simulink model "Demo_V2X_RoadWorks_cs"  (R2014b)
settings: Solver=ode5  SolverMode=SingleTasking  StartTime=0.0  StopTime=18  FixedStep=1/100  RelTol=1e-3
PreLoadFcn:
  | mbxruntime.callbacks.PreLoadFcn(bdroot);
  | check_NUTS_defined;
  | 
  | assignin('base',['model_closed_' bdroot],false);
PostLoadFcn:
  | mbxruntime.callbacks.PostLoadFcn(bdroot);
InitFcn:
  | mbxruntime.callbacks.InitFcn(bdroot);
StartFcn:
  | mbxruntime.callbacks.StartFcn(bdroot);
StopFcn:
  | mbxruntime.callbacks.StopFcn(bdroot);
model workspace: external: MAT-File .\Demo_V2X_RoadWorks_cs_hws.mat (data not in the file)
undefined symbols (not defined in the file or in its folder): InitializeBus, mbxruntime, Newton, Raphson, tabledata
undefined symbols (not defined in the file): Demo_V2X_RoadWorks_cs_002408181c311178, Demo_V2X_RoadWorks_cs_02afd40c5576fd79, Demo_V2X_RoadWorks_cs_09062d95c4976b80, Demo_V2X_RoadWorks_cs_0ad60e46608f1bfe, Demo_V2X_RoadWorks_cs_0b386a01b2cd5e8d, Demo_V2X_RoadWorks_cs_0d795afaa024d2ee, Demo_V2X_RoadWorks_cs_104085e65c337077, Demo_V2X_RoadWorks_cs_126564f7b2997a49, Demo_V2X_RoadWorks_cs_15e6e2595e8bf329, Demo_V2X_RoadWorks_cs_16adfea7655bce18, Demo_V2X_RoadWorks_cs_18ab2686f8449f50, Demo_V2X_RoadWorks_cs_1c28437def32f9f6, Demo_V2X_RoadWorks_cs_1d541c73c3d8f25b, Demo_V2X_RoadWorks_cs_1fb1f994fe012d27, Demo_V2X_RoadWorks_cs_20c117b9827230b9, Demo_V2X_RoadWorks_cs_220b1226a84e3b37, Demo_V2X_RoadWorks_cs_24814049c8ab2e18, Demo_V2X_RoadWorks_cs_24a281220a6492a7, Demo_V2X_RoadWorks_cs_279aea126b4236ad, Demo_V2X_RoadWorks_cs_28eadd0b23e572db, Demo_V2X_RoadWorks_cs_291fe7210f9ba434, Demo_V2X_RoadWorks_cs_2fd90504f8814746, Demo_V2X_RoadWorks_cs_33c1737bfc1c651f, Demo_V2X_RoadWorks_cs_388e22d5b1056b8f, Demo_V2X_RoadWorks_cs_3e3a415e868663e7, Demo_V2X_RoadWorks_cs_45759eb0c1816b1e, Demo_V2X_RoadWorks_cs_45f301cf6c396570, Demo_V2X_RoadWorks_cs_47686124f5151dea, Demo_V2X_RoadWorks_cs_487931e8a8cef1d6, Demo_V2X_RoadWorks_cs_54cb5626dca53ab7, Demo_V2X_RoadWorks_cs_56c0a253fe7e7ec0, Demo_V2X_RoadWorks_cs_5921488c0ba4168e, Demo_V2X_RoadWorks_cs_5ca0c70551eea1b3, Demo_V2X_RoadWorks_cs_5cc6ddb60eb17926, Demo_V2X_RoadWorks_cs_5dda33a127b53dd9, Demo_V2X_RoadWorks_cs_60729aca19e3b8ea, Demo_V2X_RoadWorks_cs_61616eaaf58ec115, Demo_V2X_RoadWorks_cs_63af626c9fae5224, Demo_V2X_RoadWorks_cs_649c6af7b111a61f, Demo_V2X_RoadWorks_cs_64e2df335ac415c1, Demo_V2X_RoadWorks_cs_6530f1ae727e39fe, Demo_V2X_RoadWorks_cs_6837be8d052ff1e3, Demo_V2X_RoadWorks_cs_6e8b51a123f1a201, Demo_V2X_RoadWorks_cs_6f4ec518a68cacb3, Demo_V2X_RoadWorks_cs_74dac4a6b9859226, Demo_V2X_RoadWorks_cs_75671d8cae67d5b6, Demo_V2X_RoadWorks_cs_756d40a88ae84d39, Demo_V2X_RoadWorks_cs_77c7cbc4fa1cdaa5, Demo_V2X_RoadWorks_cs_7b9fbc44403bb8f3, Demo_V2X_RoadWorks_cs_7c118b74c8d14c00, Demo_V2X_RoadWorks_cs_7c4a172761f05beb, Demo_V2X_RoadWorks_cs_80b7a78efe24d5f1, Demo_V2X_RoadWorks_cs_82d65efce1f7c4ea, Demo_V2X_RoadWorks_cs_8be5dc2565229ce9, Demo_V2X_RoadWorks_cs_8dc36f0ab6cec640, Demo_V2X_RoadWorks_cs_91305dd1362bb00d, Demo_V2X_RoadWorks_cs_929c2ffed1faf33f, Demo_V2X_RoadWorks_cs_95615bcbc0d062f1, Demo_V2X_RoadWorks_cs_99a6391a40f894df, Demo_V2X_RoadWorks_cs_9caa19175765ea5d ... (+52)
libraries: PreScanSimulinkLibrary x34, simulink_extras x15, simulink x6
(part 1 of 16)
CloseFcn:
  | mbxruntime.callbacks.CloseFcn(bdroot);
  | evalin('base',['clear model_closed_' bdroot]);
  | 
  | try
  |     close (V2x_TC_GUI)
  | end
settings Model: Creator=PRESCAN  LastModifiedBy=stq0ee
settings DataIOCC: SignalLoggingSaveFormat=ModelDataLogs
settings OptimizationCC: InlineParams=on  ExpressionDepthLimit=2147483647  InitFltsAndDblsToZero=on
settings DebuggingCC: SaveWithParameterizedLinksMsg=none  UnderspecifiedInitializationDetection=Classic  MergeDetectMultiDrivingBlocksExec=none  SignalResolutionControl=TryResolveAllWithWarning  SolverPrmCheckMsg=none  MultiTaskDSMMsg=warning  MultiTaskCondExecSysMsg=none  FcnCallInpInsideContextMsg=UseLocalSettings  StateNameClashWarn=warning
settings ModelReferenceCC: UpdateModelReferenceTargets=IfOutOfDate
settings SFSimCC: SimParseCustomCode=off
settings SFSimCC: SimCustomHeaderCode=|
  | #include "prescan.h"
  | #include "prescan_platform.h"
  | #include "prescan_v2x_data.h"
settings RTWCC: IncludeERTFirstTime=on
settings GRTTargetCC: TargetFcnLib=ansi_tfl_tmw.mat  CombineOutputUpdateFcns=off  GRTInterface=on

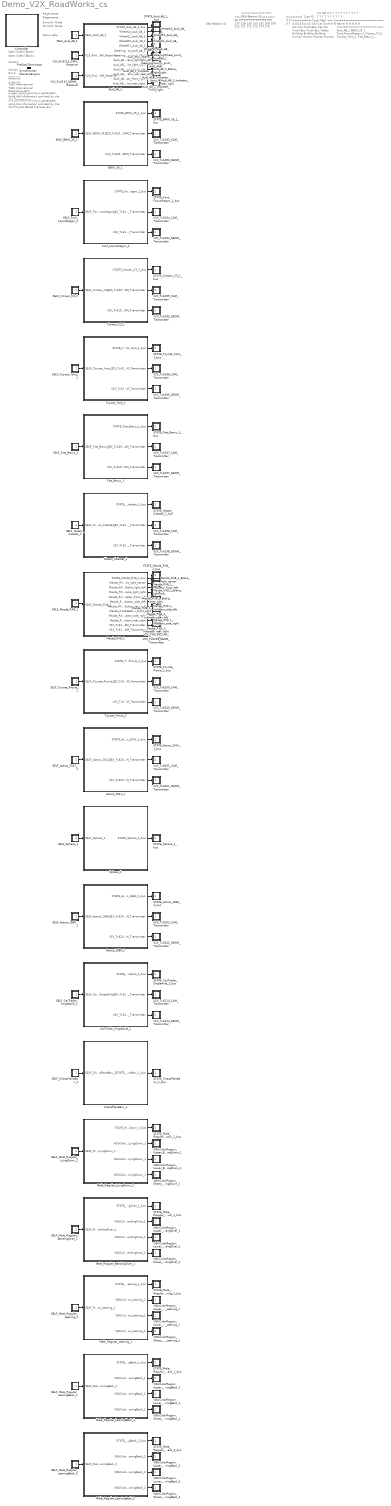
== system Demo_V2X_RoadWorks_cs ==
  note: Regenerate
  note: Simulink Mode
  note: Open Useful Blocks
  note: 2020.1.0
  note: Version:
  note: Author(s):
  note: TASS International
  note: Descriptive text:
  note: A road works warning is generated
      | using the information provided by
      | the V2X Physics Based Transceivers.
  note: OBU-Beacon ID
  note: Demo Help
  note: 8.6.0
  note: A road works warning is generated
      | using the information provided by
      | the V2X Transceivers.
  note: Descriptive text:
  note: TASS International
  note: Author(s):
  note: Version:
  note: Open Useful Blocks
  note: Simulink Mode
  note: Regenerate
  note: ======
      | Num ID
      | ======
      | 36
      | 95
      | 130
      | 131
      | 132
      | 133
      | 135
      | 137
      | 138
      | 139
      | 153
      | 152
      | 208
      | 209
      | 212
      | 171
      | 172
      | 173
      | 174
      | 175
  note: =============
      | OBU-Beacon ID
      | =============
  note: =======
      | Type ID
      | =======
      | 1
      | 1
      | 1
      | 1
      | 1
      | 1
      | 3
      | 1
      | 1
      | 3
      | 3
      | 7
      | 12
      | 12
      | 12
      | 4
      | 4
      | 4
      | 4
      | 4
  note: ========
      | Type Tag
      | ========
      | Car
      | Car
      | Car
      | Car
      | Car
      | Car
      | Truck\Bus
      | Car
      | Car
      | Truck\Bus
      | Truck\Bus
      | Trailer
      | Building
      | Building
      | Building
      | Human
      | Human
      | Human
      | Human
      | Human
  note: ==
      | SD
      | ==
      | Y
      | Y
      | Y
      | Y
      | Y
      | Y
      | Y
      | Y
      | Y
      | Y
      | Y
      | Y
      | Y
      | Y
      | Y
      | Y
      | Y
      | Y
      | Y
      | Y
  note: ==
      | CD
      | ==
      | N
      | N
      | N
      | N
      | N
      | N
      | N
      | N
      | N
      | N
      | N
      | N
      | N
      | N
      | N
      | N
      | N
      | N
      | N
      | N
  note: ====================
      | Name
      | ====================
      | Audi_A8_1
      | BMW_X5_1
      | Ford_FocusWagon_1
      | Citroen_C3_1
      | Toyota_Yaris_1
      | Fiat_Bravo_1
      | Nissan_Cabstar_1
      | Mazda_RX8_1
      | Toyota_Previa_1
      | Actros_2541_1
      | Actros_1860_1
      | CarTrailer_SingleAxle_1
      | GasStation_1
      | Warehouse_1
      | Windmill_1
      | Male_Regular_LyingDown_1
      | Male_Regular_BendingOver_1
      | Male_Regular_Leaning_1
      | Male_Regular_LeaningBack_1
      | Male_Regular_LeaningBack_2
  Actros_1860_1 : Subsystem  Tag=WorldObjectSubSystem  InitFcn=UniqueId = '3711';
      mask init:
      | modelPath = GenericModelHelper.getGenericModelFilePath('ModelDepo','Vehicles\Mercedes_Actros_1860\Mercedes_Actros_1860.pgmb','f4d262a59d21672e46677209b578f5e0');imagePath = GenericModelHelper.getCompilationPicture(modelPath, 'Mercedes_Actros_1860_HighPoly.png');
      mask Display: image(imread(imagePath));color('white');text(0, 0, ' ID=153\n')
  Actros_2541_1 : Subsystem  Tag=WorldObjectSubSystem  InitFcn=UniqueId = '3609';
      mask init:
      | modelPath = GenericModelHelper.getGenericModelFilePath('ModelDepo','Vehicles\Mercedes_Actros_2541\Mercedes_Actros_2541.pgmb','2272788c542945e1b586df6742792b5a');imagePath = GenericModelHelper.getCompilationPicture(modelPath, 'Mercedes_Actros_2541_HighPoly.png');
      mask Display: image(imread(imagePath));color('white');text(0, 0, ' ID=139\n')
  Audi_A8_1 : Subsystem  Tag=WorldObjectSubSystem  InitFcn=UniqueId = '1227';
      mask init:
      | modelPath = GenericModelHelper.getGenericModelFilePath('ModelDepo','Vehicles\Audi_A8\Audi_A8.pgmb','e33fe1ddcf3e8ae97caccbc8f2fa74ac');imagePath = GenericModelHelper.getCompilationPicture(modelPath, 'Audi_A8_HighPoly.png');
      mask Display: image(imread(imagePath));color('white');text(0, 0, ' ID=36\n')
  Audi_A8_1_Brake_light_left : Subsystem  Tag=actuator/BrakeLightL  Priority=0  LoadFcn=load('PreScanVisuLightActuatorData');load('PrescanRPYData');load('PrescanXYZData');load('PreScanRGBData')  mask(PreScan Sink Block: VisuActiveLight){}
      mask help:
      | The VisuActiveLight block provides a way for detailed animation of Light Sources, such as the indicator, brake, fog and main lights of a vehicle, or a light post.
      |
      | For more information, please click Help.
      settings: OpenFcn=open_system([gcb '/Actuator'],'mask')
      mask Help: eval('openHelp(209)')
      mask Display: image(imread('HeadLight.png'))
  Audi_A8_1_Brake_light_right : Subsystem  Tag=actuator/BrakeLightR  Priority=0  LoadFcn=load('PreScanVisuLightActuatorData');load('PrescanRPYData');load('PrescanXYZData');load('PreScanRGBData')  mask(PreScan Sink Block: VisuActiveLight){}
      mask help:
      | The VisuActiveLight block provides a way for detailed animation of Light Sources, such as the indicator, brake, fog and main lights of a vehicle, or a light post.
      |
      | For more information, please click Help.
      settings: OpenFcn=open_system([gcb '/Actuator'],'mask')
      mask Help: eval('openHelp(209)')
      mask Display: image(imread('HeadLight.png'))
  Audi_A8_1_Indicator_front_left : Subsystem  Tag=actuator/IndicatorFL  Priority=0  LoadFcn=load('PreScanVisuLightActuatorData');load('PrescanRPYData');load('PrescanXYZData');load('PreScanRGBData')  mask(PreScan Sink Block: VisuActiveLight){}
      mask help:
      | The VisuActiveLight block provides a way for detailed animation of Light Sources, such as the indicator, brake, fog and main lights of a vehicle, or a light post.
      |
      | For more information, please click Help.
      settings: OpenFcn=open_system([gcb '/Actuator'],'mask')
      mask Help: eval('openHelp(209)')
      mask Display: image(imread('HeadLight.png'))
  Audi_A8_1_Indicator_front_right : Subsystem  Tag=actuator/IndicatorFR  Priority=0  LoadFcn=load('PreScanVisuLightActuatorData');load('PrescanRPYData');load('PrescanXYZData');load('PreScanRGBData')  mask(PreScan Sink Block: VisuActiveLight){}
      mask help:
      | The VisuActiveLight block provides a way for detailed animation of Light Sources, such as the indicator, brake, fog and main lights of a vehicle, or a light post.
      |
      | For more information, please click Help.
      settings: OpenFcn=open_system([gcb '/Actuator'],'mask')
      mask Help: eval('openHelp(209)')
      mask Display: image(imread('HeadLight.png'))
  Audi_A8_1_Indicator_rear_left : Subsystem  Tag=actuator/IndicatorRL  Priority=0  LoadFcn=load('PreScanVisuLightActuatorData');load('PrescanRPYData');load('PrescanXYZData');load('PreScanRGBData')  mask(PreScan Sink Block: VisuActiveLight){}
      mask help:
      | The VisuActiveLight block provides a way for detailed animation of Light Sources, such as the indicator, brake, fog and main lights of a vehicle, or a light post.
      |
      | For more information, please click Help.
      settings: OpenFcn=open_system([gcb '/Actuator'],'mask')
      mask Help: eval('openHelp(209)')
      mask Display: image(imread('HeadLight.png'))
  Audi_A8_1_Indicator_rear_right : Subsystem  Tag=actuator/IndicatorRR  Priority=0  LoadFcn=load('PreScanVisuLightActuatorData');load('PrescanRPYData');load('PrescanXYZData');load('PreScanRGBData')  mask(PreScan Sink Block: VisuActiveLight){}
      mask help:
      | The VisuActiveLight block provides a way for detailed animation of Light Sources, such as the indicator, brake, fog and main lights of a vehicle, or a light post.
      |
      | For more information, please click Help.
      settings: OpenFcn=open_system([gcb '/Actuator'],'mask')
      mask Help: eval('openHelp(209)')
      mask Display: image(imread('HeadLight.png'))
  BMW_X5_1 : Subsystem  Tag=WorldObjectSubSystem  InitFcn=UniqueId = '3531';
      mask init:
      | modelPath = GenericModelHelper.getGenericModelFilePath('ModelDepo','Vehicles\BMW_X5\BMW_X5.pgmb','bfeb1c11467705ab888b3011684c848b');imagePath = GenericModelHelper.getCompilationPicture(modelPath, 'BMW_X5_HighPoly.png');
      mask Display: image(imread(imagePath));color('white');text(0, 0, ' ID=95\n')
  CarTrailer_SingleAxle_1 : Subsystem  Tag=WorldObjectSubSystem  InitFcn=UniqueId = '4026';
      mask init:
      | modelPath = GenericModelHelper.getGenericModelFilePath('ModelDepo','Vehicles\Car_Trailer\Car_Trailer.pgmb','78eb1271f3472dc97c9b4c36c623cf76');imagePath = GenericModelHelper.getCompilationPicture(modelPath, 'Car_Trailer_HighPoly.png');
      mask Display: image(imread(imagePath));color('white');text(0, 0, ' ID=152\n')
  ChessPlaneBox_1 : Subsystem  Tag=WorldObjectSubSystem  InitFcn=UniqueId = '4034';
      mask init:
      | imagePath=which('ChessPlaneBox.jpg');
      mask Display: image(imread(imagePath));color('white');text(0, 0, ' ID=177\n')
  Citroen_C3_1 : Subsystem  Tag=WorldObjectSubSystem  InitFcn=UniqueId = '3533';
      mask init:
      | modelPath = GenericModelHelper.getGenericModelFilePath('ModelDepo','Vehicles\Citroen_C3\Citroen_C3.pgmb','e804ced06d50dbfc6a2202ab3ad01b0c');imagePath = GenericModelHelper.getCompilationPicture(modelPath, 'Citroen_C3_HighPoly.png');
      mask Display: image(imread(imagePath));color('white');text(0, 0, ' ID=131\n')
  Controller : Subsystem  Description=8A3CD2955739A82C886C20AE3E253D78460D53180EE2C1B14CC08DF75A70BE77  Priority=-1  LoadFcn=load PreScanControllerData  mask(PreScan Simulation Controller){prescanversion='2020.1.0', ModelReferencing=off, TimeStep=1/100, ControlMode=0, PreScanExecutionMode=on, ControllerCount=0, ControllerIndex=0, ControllerOptions=''}
      mask prompts: prescanversion "PreScan Version"; ModelReferencing "Use Model Referencing"; TimeStep "Upload Period [s]"; ControlMode "Control Mode"; PreScanExecutionMode "Execution Mode"; ControllerCount "Controller Count"; ControllerIndex "Controller Index"; ControllerOptions "Controller Options"
      mask help:
      | Please do not remove this block from the compilation sheet,
      | as it connects the model to the PreScan environment.
      mask init:
      | model = bdroot(gcb);
      | ExperimentFile = mbxruntime.findExperimentFile(model,true); %relative path
      | 
      | [d1, d2, d3, prescandata] = prescan_Settings();
      | ModelDepo = fullfile(prescandata,'ModelDepo'); 
      | 
      | RTmode = mbxruntime.getRTMode(model);
      | 
      | SimulationMode = get_param(bdroot,'SimulationMode');
      | if strcmp(SimulationMode, 'rapid-accelerator')
      |     SimulationMode = 'external';
      | end
      | TargetName = get_param(bdroot,'SystemTargetFile');
      settings: ModelCloseFcn=assignin('base',['model_closed_' bdroot],true);
      mask Help: eval('openHelp(812)')
      mask Display: image(imread('prescanlogo.ico'))
  Fiat_Bravo_1 : Subsystem  Tag=WorldObjectSubSystem  InitFcn=UniqueId = '3535';
      mask init:
      | modelPath = GenericModelHelper.getGenericModelFilePath('ModelDepo','Vehicles\Fiat_Bravo\Fiat_Bravo.pgmb','a97eb0ec4093646e5d079d2ab9a2eab7');imagePath = GenericModelHelper.getCompilationPicture(modelPath, 'Fiat_Bravo_HighPoly.png');
      mask Display: image(imread(imagePath));color('white');text(0, 0, ' ID=133\n')
  Ford_FocusWagon_1 : Subsystem  Tag=WorldObjectSubSystem  InitFcn=UniqueId = '3532';
      mask init:
      | modelPath = GenericModelHelper.getGenericModelFilePath('ModelDepo','Vehicles\Ford_Focus_Wagon\Ford_Focus_Wagon.pgmb','b2649206ae23d0f1e06c4f4bbfea8272');imagePath = GenericModelHelper.getCompilationPicture(modelPath, 'Ford_Focus_Wagon_HighPoly.png');
      mask Display: image(imread(imagePath));color('white');text(0, 0, ' ID=130\n')
  Male_Regular_BendingOver_1 : Subsystem  Tag=WorldObjectSubSystem  InitFcn=UniqueId = '4029';
      mask init:
      | modelPath = GenericModelHelper.getGenericModelFilePath('ModelDepo','Humans\MaleBendingOver\Male_BendingOver.pgmb','cef88e240e9b911a86b5636bd81955cf');imagePath = GenericModelHelper.getCompilationPicture(modelPath, 'MaleBendingOver.png');
      mask Display: image(imread(imagePath));color('white');text(0, 0, ' ID=172\n')
  Male_Regular_LeaningBack_1 : Subsystem  Tag=WorldObjectSubSystem  InitFcn=UniqueId = '4031';
      mask init:
      | modelPath = GenericModelHelper.getGenericModelFilePath('ModelDepo','Humans\MaleLeaningBack\Male_LeaningBack.pgmb','135846bff650550b8f28a3f3fa1bf4a5');imagePath = GenericModelHelper.getCompilationPicture(modelPath, 'MaleLeaningBack.png');
      mask Display: image(imread(imagePath));color('white');text(0, 0, ' ID=174\n')
  Male_Regular_LeaningBack_2 : Subsystem  Tag=WorldObjectSubSystem  InitFcn=UniqueId = '4032';
      mask init: same as Demo_V2X_RoadWorks_cs/Male_Regular_LeaningBack_1
      mask Display: image(imread(imagePath));color('white');text(0, 0, ' ID=175\n')
  Male_Regular_Leaning_1 : Subsystem  Tag=WorldObjectSubSystem  InitFcn=UniqueId = '4030';
      mask init:
      | modelPath = GenericModelHelper.getGenericModelFilePath('ModelDepo','Humans\MaleLeaning\Male_Leaning.pgmb','25c16c562fbaf9d24ccaeafbcaf6911f');imagePath = GenericModelHelper.getCompilationPicture(modelPath, 'MaleLeaning.png');
      mask Display: image(imread(imagePath));color('white');text(0, 0, ' ID=173\n')
  Male_Regular_LyingDown_1 : Subsystem  Tag=WorldObjectSubSystem  InitFcn=UniqueId = '4028';
      mask init:
      | modelPath = GenericModelHelper.getGenericModelFilePath('ModelDepo','Humans\MaleLyingDown\Male_LyingDown.pgmb','1d218d8ab2130673bd658bb3c3249a51');imagePath = GenericModelHelper.getCompilationPicture(modelPath, 'MaleLyingDown.png');
      mask Display: image(imread(imagePath));color('white');text(0, 0, ' ID=171\n')
  Mazda_RX8_1 : Subsystem  Tag=WorldObjectSubSystem  InitFcn=UniqueId = '3607';
      mask init:
      | modelPath = GenericModelHelper.getGenericModelFilePath('ModelDepo','Vehicles\Mazda_RX8\Mazda_RX8.pgmb','1e55a2e40efa576b7f4fb93bae35d605');imagePath = GenericModelHelper.getCompilationPicture(modelPath, 'Mazda_RX8_HighPoly.png');
      mask Display: image(imread(imagePath));color('white');text(0, 0, ' ID=137\n')
  Mazda_RX8_1_Brake_light_center : Subsystem  Tag=actuator/BrakeLightM  Priority=0  LoadFcn=load('PreScanVisuLightActuatorData');load('PrescanRPYData');load('PrescanXYZData');load('PreScanRGBData')  mask(PreScan Sink Block: VisuActiveLight){}
      mask help:
      | The VisuActiveLight block provides a way for detailed animation of Light Sources, such as the indicator, brake, fog and main lights of a vehicle, or a light post.
      |
      | For more information, please click Help.
      settings: OpenFcn=open_system([gcb '/Actuator'],'mask')
      mask Help: eval('openHelp(209)')
      mask Display: image(imread('HeadLight.png'))
  Mazda_RX8_1_Brake_light_left : Subsystem  Tag=actuator/BrakeLightL  Priority=0  LoadFcn=load('PreScanVisuLightActuatorData');load('PrescanRPYData');load('PrescanXYZData');load('PreScanRGBData')  mask(PreScan Sink Block: VisuActiveLight){}
      mask help:
      | The VisuActiveLight block provides a way for detailed animation of Light Sources, such as the indicator, brake, fog and main lights of a vehicle, or a light post.
      |
      | For more information, please click Help.
      settings: OpenFcn=open_system([gcb '/Actuator'],'mask')
      mask Help: eval('openHelp(209)')
      mask Display: image(imread('HeadLight.png'))
  Mazda_RX8_1_Brake_light_right : Subsystem  Tag=actuator/BrakeLightR  Priority=0  LoadFcn=load('PreScanVisuLightActuatorData');load('PrescanRPYData');load('PrescanXYZData');load('PreScanRGBData')  mask(PreScan Sink Block: VisuActiveLight){}
      mask help:
      | The VisuActiveLight block provides a way for detailed animation of Light Sources, such as the indicator, brake, fog and main lights of a vehicle, or a light post.
      |
      | For more information, please click Help.
      settings: OpenFcn=open_system([gcb '/Actuator'],'mask')
      mask Help: eval('openHelp(209)')
      mask Display: image(imread('HeadLight.png'))
  Mazda_RX8_1_Indicator_front_left : Subsystem  Tag=actuator/IndicatorFL  Priority=0  LoadFcn=load('PreScanVisuLightActuatorData');load('PrescanRPYData');load('PrescanXYZData');load('PreScanRGBData')  mask(PreScan Sink Block: VisuActiveLight){}
      mask help:
      | The VisuActiveLight block provides a way for detailed animation of Light Sources, such as the indicator, brake, fog and main lights of a vehicle, or a light post.
      |
      | For more information, please click Help.
      settings: OpenFcn=open_system([gcb '/Actuator'],'mask')
      mask Help: eval('openHelp(209)')
      mask Display: image(imread('HeadLight.png'))
  Mazda_RX8_1_Indicator_front_right : Subsystem  Tag=actuator/IndicatorFR  Priority=0  LoadFcn=load('PreScanVisuLightActuatorData');load('PrescanRPYData');load('PrescanXYZData');load('PreScanRGBData')  mask(PreScan Sink Block: VisuActiveLight){}
      mask help:
      | The VisuActiveLight block provides a way for detailed animation of Light Sources, such as the indicator, brake, fog and main lights of a vehicle, or a light post.
      |
      | For more information, please click Help.
      settings: OpenFcn=open_system([gcb '/Actuator'],'mask')
      mask Help: eval('openHelp(209)')
      mask Display: image(imread('HeadLight.png'))
  Mazda_RX8_1_Indicator_rear_left : Subsystem  Tag=actuator/IndicatorRL  Priority=0  LoadFcn=load('PreScanVisuLightActuatorData');load('PrescanRPYData');load('PrescanXYZData');load('PreScanRGBData')  mask(PreScan Sink Block: VisuActiveLight){}
      mask help:
      | The VisuActiveLight block provides a way for detailed animation of Light Sources, such as the indicator, brake, fog and main lights of a vehicle, or a light post.
      |
      | For more information, please click Help.
      settings: OpenFcn=open_system([gcb '/Actuator'],'mask')
      mask Help: eval('openHelp(209)')
      mask Display: image(imread('HeadLight.png'))
  Mazda_RX8_1_Indicator_rear_right : Subsystem  Tag=actuator/IndicatorRR  Priority=0  LoadFcn=load('PreScanVisuLightActuatorData');load('PrescanRPYData');load('PrescanXYZData');load('PreScanRGBData')  mask(PreScan Sink Block: VisuActiveLight){}
      mask help:
      | The VisuActiveLight block provides a way for detailed animation of Light Sources, such as the indicator, brake, fog and main lights of a vehicle, or a light post.
      |
      | For more information, please click Help.
      settings: OpenFcn=open_system([gcb '/Actuator'],'mask')
      mask Help: eval('openHelp(209)')
      mask Display: image(imread('HeadLight.png'))
  Mazda_RX8_1_Indicator_side_left : Subsystem  Tag=actuator/IndicatorSL  Priority=0  LoadFcn=load('PreScanVisuLightActuatorData');load('PrescanRPYData');load('PrescanXYZData');load('PreScanRGBData')  mask(PreScan Sink Block: VisuActiveLight){}
      mask help:
      | The VisuActiveLight block provides a way for detailed animation of Light Sources, such as the indicator, brake, fog and main lights of a vehicle, or a light post.
      |
      | For more information, please click Help.
      settings: OpenFcn=open_system([gcb '/Actuator'],'mask')
      mask Help: eval('openHelp(209)')
      mask Display: image(imread('HeadLight.png'))
  Mazda_RX8_1_Indicator_side_right : Subsystem  Tag=actuator/IndicatorSR  Priority=0  LoadFcn=load('PreScanVisuLightActuatorData');load('PrescanRPYData');load('PrescanXYZData');load('PreScanRGBData')  mask(PreScan Sink Block: VisuActiveLight){}
      mask help:
      | The VisuActiveLight block provides a way for detailed animation of Light Sources, such as the indicator, brake, fog and main lights of a vehicle, or a light post.
      |
      | For more information, please click Help.
      settings: OpenFcn=open_system([gcb '/Actuator'],'mask')
      mask Help: eval('openHelp(209)')
      mask Display: image(imread('HeadLight.png'))
  Nissan_Cabstar_1 : Subsystem  Tag=WorldObjectSubSystem  InitFcn=UniqueId = '3606';
      mask init:
      | modelPath = GenericModelHelper.getGenericModelFilePath('ModelDepo','Vehicles\Nissan_Cabstar\Nissan_Cabstar.pgmb','dd076fdae311093c5436e82e6c23dc23');imagePath = GenericModelHelper.getCompilationPicture(modelPath, 'Nissan_Cabstar_HighPoly.png');
      mask Display: image(imread(imagePath));color('white');text(0, 0, ' ID=135\n')
  PreScanTerminator : Subsystem  Tag=PreScanTerminator  Priority=999  LoadFcn=load PrescanTerminatorData  mask(PreScan Simulation Terminator){TimeStep=1/100}
      mask prompts: TimeStep "Upload Period [s]"
      mask help:
      | Please do not remove this block from the compilation sheet as it
      | connects the model to the PreScan environment.
      mask Help: eval('openHelp(812)')
      mask Display: image(imread('prescanlogo.ico'))
  SELF_Actros_1860_1 : Subsystem  Tag=sensor/SelfPort  Priority=30  LoadFcn=load('PreScanSelfSensorData.mat')  mask(PreScan Source Block: SELF){}
      mask help:
      | The SELF port shows (state) information of the actor itself. The outputs are position in the experiment's axis system and the GPS coordinates, and the object's absolute velocity and compass heading.
      |
      | For more information, please click Help.
      settings: OpenFcn=open_system([gcb '/Sensor'],'mask')
      mask Help: eval('openHelp(462)')
      mask Display: image(imread('GPS.png'))
  SELF_Actros_2541_1 : Subsystem  Tag=sensor/SelfPort  Priority=30  LoadFcn=load('PreScanSelfSensorData.mat')  mask(PreScan Source Block: SELF){}
      mask help:
      | The SELF port shows (state) information of the actor itself. The outputs are position in the experiment's axis system and the GPS coordinates, and the object's absolute velocity and compass heading.
      |
      | For more information, please click Help.
      settings: OpenFcn=open_system([gcb '/Sensor'],'mask')
      mask Help: eval('openHelp(462)')
      mask Display: image(imread('GPS.png'))
  SELF_Audi_A8_1 : Subsystem  Tag=sensor/SelfPort  Priority=30  LoadFcn=load('PreScanSelfSensorData.mat')  mask(PreScan Source Block: SELF){}
      mask help:
      | The SELF port shows (state) information of the actor itself. The outputs are position in the experiment's axis system and the GPS coordinates, and the object's absolute velocity and compass heading.
      |
      | For more information, please click Help.
      settings: OpenFcn=open_system([gcb '/Sensor'],'mask')
      mask Help: eval('openHelp(462)')
      mask Display: image(imread('GPS.png'))
  SELF_BMW_X5_1 : Subsystem  Tag=sensor/SelfPort  Priority=30  LoadFcn=load('PreScanSelfSensorData.mat')  mask(PreScan Source Block: SELF){}
      mask help:
      | The SELF port shows (state) information of the actor itself. The outputs are position in the experiment's axis system and the GPS coordinates, and the object's absolute velocity and compass heading.
      |
      | For more information, please click Help.
      settings: OpenFcn=open_system([gcb '/Sensor'],'mask')
      mask Help: eval('openHelp(462)')
      mask Display: image(imread('GPS.png'))
  SELF_CarTrailer_SingleAxle_1 : Subsystem  Tag=sensor/SelfPort  Priority=30  LoadFcn=load('PreScanSelfSensorData.mat')  mask(PreScan Source Block: SELF){}
      mask help:
      | The SELF port shows (state) information of the actor itself. The outputs are position in the experiment's axis system and the GPS coordinates, and the object's absolute velocity and compass heading.
      |
      | For more information, please click Help.
      settings: OpenFcn=open_system([gcb '/Sensor'],'mask')
      mask Help: eval('openHelp(462)')
      mask Display: image(imread('GPS.png'))
  SELF_ChessPlaneBox_1 : Subsystem  Tag=sensor/SelfPort  Priority=30  LoadFcn=load('PreScanSelfSensorData.mat')  mask(PreScan Source Block: SELF){}
      mask help:
      | The SELF port shows (state) information of the actor itself. The outputs are position in the experiment's axis system and the GPS coordinates, and the object's absolute velocity and compass heading.
      |
      | For more information, please click Help.
      settings: OpenFcn=open_system([gcb '/Sensor'],'mask')
      mask Help: eval('openHelp(462)')
      mask Display: image(imread('GPS.png'))
  SELF_Citroen_C3_1 : Subsystem  Tag=sensor/SelfPort  Priority=30  LoadFcn=load('PreScanSelfSensorData.mat')  mask(PreScan Source Block: SELF){}
      mask help:
      | The SELF port shows (state) information of the actor itself. The outputs are position in the experiment's axis system and the GPS coordinates, and the object's absolute velocity and compass heading.
      |
      | For more information, please click Help.
      settings: OpenFcn=open_system([gcb '/Sensor'],'mask')
      mask Help: eval('openHelp(462)')
      mask Display: image(imread('GPS.png'))
  SELF_Fiat_Bravo_1 : Subsystem  Tag=sensor/SelfPort  Priority=30  LoadFcn=load('PreScanSelfSensorData.mat')  mask(PreScan Source Block: SELF){}
      mask help:
      | The SELF port shows (state) information of the actor itself. The outputs are position in the experiment's axis system and the GPS coordinates, and the object's absolute velocity and compass heading.
      |
      | For more information, please click Help.
      settings: OpenFcn=open_system([gcb '/Sensor'],'mask')
      mask Help: eval('openHelp(462)')
      mask Display: image(imread('GPS.png'))
  SELF_Ford_FocusWagon_1 : Subsystem  Tag=sensor/SelfPort  Priority=30  LoadFcn=load('PreScanSelfSensorData.mat')  mask(PreScan Source Block: SELF){}
      mask help:
      | The SELF port shows (state) information of the actor itself. The outputs are position in the experiment's axis system and the GPS coordinates, and the object's absolute velocity and compass heading.
      |
      | For more information, please click Help.
      settings: OpenFcn=open_system([gcb '/Sensor'],'mask')
      mask Help: eval('openHelp(462)')
      mask Display: image(imread('GPS.png'))
  SELF_Male_Regular_BendingOver_1 : Subsystem  Tag=sensor/SelfPort  Priority=30  LoadFcn=load('PreScanSelfSensorData.mat')  mask(PreScan Source Block: SELF){}
      mask help:
      | The SELF port shows (state) information of the actor itself. The outputs are position in the experiment's axis system and the GPS coordinates, and the object's absolute velocity and compass heading.
      |
      | For more information, please click Help.
      settings: OpenFcn=open_system([gcb '/Sensor'],'mask')
      mask Help: eval('openHelp(462)')
      mask Display: image(imread('GPS.png'))
  SELF_Male_Regular_LeaningBack_1 : Subsystem  Tag=sensor/SelfPort  Priority=30  LoadFcn=load('PreScanSelfSensorData.mat')  mask(PreScan Source Block: SELF){}
      mask help:
      | The SELF port shows (state) information of the actor itself. The outputs are position in the experiment's axis system and the GPS coordinates, and the object's absolute velocity and compass heading.
      |
      | For more information, please click Help.
      settings: OpenFcn=open_system([gcb '/Sensor'],'mask')
      mask Help: eval('openHelp(462)')
      mask Display: image(imread('GPS.png'))
  SELF_Male_Regular_LeaningBack_2 : Subsystem  Tag=sensor/SelfPort  Priority=30  LoadFcn=load('PreScanSelfSensorData.mat')  mask(PreScan Source Block: SELF){}
      mask help:
      | The SELF port shows (state) information of the actor itself. The outputs are position in the experiment's axis system and the GPS coordinates, and the object's absolute velocity and compass heading.
      |
      | For more information, please click Help.
      settings: OpenFcn=open_system([gcb '/Sensor'],'mask')
      mask Help: eval('openHelp(462)')
      mask Display: image(imread('GPS.png'))
  SELF_Male_Regular_Leaning_1 : Subsystem  Tag=sensor/SelfPort  Priority=30  LoadFcn=load('PreScanSelfSensorData.mat')  mask(PreScan Source Block: SELF){}
      mask help:
      | The SELF port shows (state) information of the actor itself. The outputs are position in the experiment's axis system and the GPS coordinates, and the object's absolute velocity and compass heading.
      |
      | For more information, please click Help.
      settings: OpenFcn=open_system([gcb '/Sensor'],'mask')
      mask Help: eval('openHelp(462)')
      mask Display: image(imread('GPS.png'))
  SELF_Male_Regular_LyingDown_1 : Subsystem  Tag=sensor/SelfPort  Priority=30  LoadFcn=load('PreScanSelfSensorData.mat')  mask(PreScan Source Block: SELF){}
      mask help:
      | The SELF port shows (state) information of the actor itself. The outputs are position in the experiment's axis system and the GPS coordinates, and the object's absolute velocity and compass heading.
      |
      | For more information, please click Help.
      settings: OpenFcn=open_system([gcb '/Sensor'],'mask')
      mask Help: eval('openHelp(462)')
      mask Display: image(imread('GPS.png'))
  SELF_Mazda_RX8_1 : Subsystem  Tag=sensor/SelfPort  Priority=30  LoadFcn=load('PreScanSelfSensorData.mat')  mask(PreScan Source Block: SELF){}
      mask help:
      | The SELF port shows (state) information of the actor itself. The outputs are position in the experiment's axis system and the GPS coordinates, and the object's absolute velocity and compass heading.
      |
      | For more information, please click Help.
      settings: OpenFcn=open_system([gcb '/Sensor'],'mask')
      mask Help: eval('openHelp(462)')
      mask Display: image(imread('GPS.png'))
  SELF_Nissan_Cabstar_1 : Subsystem  Tag=sensor/SelfPort  Priority=30  LoadFcn=load('PreScanSelfSensorData.mat')  mask(PreScan Source Block: SELF){}
      mask help:
      | The SELF port shows (state) information of the actor itself. The outputs are position in the experiment's axis system and the GPS coordinates, and the object's absolute velocity and compass heading.
      |
      | For more information, please click Help.
      settings: OpenFcn=open_system([gcb '/Sensor'],'mask')
      mask Help: eval('openHelp(462)')
      mask Display: image(imread('GPS.png'))
  SELF_Sphere_1 : Subsystem  Tag=sensor/SelfPort  Priority=30  LoadFcn=load('PreScanSelfSensorData.mat')  mask(PreScan Source Block: SELF){}
      mask help:
      | The SELF port shows (state) information of the actor itself. The outputs are position in the experiment's axis system and the GPS coordinates, and the object's absolute velocity and compass heading.
      |
      | For more information, please click Help.
      settings: OpenFcn=open_system([gcb '/Sensor'],'mask')
      mask Help: eval('openHelp(462)')
      mask Display: image(imread('GPS.png'))
  SELF_Toyota_Previa_1 : Subsystem  Tag=sensor/SelfPort  Priority=30  LoadFcn=load('PreScanSelfSensorData.mat')  mask(PreScan Source Block: SELF){}
      mask help:
      | The SELF port shows (state) information of the actor itself. The outputs are position in the experiment's axis system and the GPS coordinates, and the object's absolute velocity and compass heading.
      |
      | For more information, please click Help.
      settings: OpenFcn=open_system([gcb '/Sensor'],'mask')
      mask Help: eval('openHelp(462)')
      mask Display: image(imread('GPS.png'))
  SELF_Toyota_Yaris_1 : Subsystem  Tag=sensor/SelfPort  Priority=30  LoadFcn=load('PreScanSelfSensorData.mat')  mask(PreScan Source Block: SELF){}
      mask help:
      | The SELF port shows (state) information of the actor itself. The outputs are position in the experiment's axis system and the GPS coordinates, and the object's absolute velocity and compass heading.
      |
      | For more information, please click Help.
      settings: OpenFcn=open_system([gcb '/Sensor'],'mask')
      mask Help: eval('openHelp(462)')
      mask Display: image(imread('GPS.png'))
  STATE_Actros_1860_1_bus : Subsystem  Tag=actuator/StatePort  Priority=0  LoadFcn=load('PreScanStateActuatorData.mat')  mask(PreScan Sink Block: State){}
      mask help:
      | The Actor State contains a vector signal of size (9x1), containing the following signals:
      |
      | -  Position    	(x,y,z)             	[m]
      | -  Velocity    	(vx,vy,vz)         	[m/s]
      | -  Angles       	(Roll, Pitch, Yaw)	[rad]
      |
      | The Actor state is defined in the global axis system.
      | The state is superponed on the Initial position defined in the GUI.
      |
      | For more information, please click Help.
      settings: OpenFcn=open_system([gcb '/Actuator'],'mask')
      mask Help: eval('openHelp(222)')
      mask Display: image(imread('State.png'))
  STATE_Actros_2541_1_bus : Subsystem  Tag=actuator/StatePort  Priority=0  LoadFcn=load('PreScanStateActuatorData.mat')  mask(PreScan Sink Block: State){}
      mask help:
      | The Actor State contains a vector signal of size (9x1), containing the following signals:
      |
      | -  Position    	(x,y,z)             	[m]
      | -  Velocity    	(vx,vy,vz)         	[m/s]
      | -  Angles       	(Roll, Pitch, Yaw)	[rad]
      |
      | The Actor state is defined in the global axis system.
      | The state is superponed on the Initial position defined in the GUI.
      |
      | For more information, please click Help.
      settings: OpenFcn=open_system([gcb '/Actuator'],'mask')
      mask Help: eval('openHelp(222)')
      mask Display: image(imread('State.png'))
  STATE_Audi_A8_1_bus : Subsystem  Tag=actuator/StatePort  Priority=0  LoadFcn=load('PreScanStateActuatorData.mat')  mask(PreScan Sink Block: State){}
      mask help:
      | The Actor State contains a vector signal of size (9x1), containing the following signals:
      |
      | -  Position    	(x,y,z)             	[m]
      | -  Velocity    	(vx,vy,vz)         	[m/s]
      | -  Angles       	(Roll, Pitch, Yaw)	[rad]
      |
      | The Actor state is defined in the global axis system.
      | The state is superponed on the Initial position defined in the GUI.
      |
      | For more information, please click Help.
      settings: OpenFcn=open_system([gcb '/Actuator'],'mask')
      mask Help: eval('openHelp(222)')
      mask Display: image(imread('State.png'))
  STATE_BMW_X5_1_bus : Subsystem  Tag=actuator/StatePort  Priority=0  LoadFcn=load('PreScanStateActuatorData.mat')  mask(PreScan Sink Block: State){}
      mask help:
      | The Actor State contains a vector signal of size (9x1), containing the following signals:
      |
      | -  Position    	(x,y,z)             	[m]
      | -  Velocity    	(vx,vy,vz)         	[m/s]
      | -  Angles       	(Roll, Pitch, Yaw)	[rad]
      |
      | The Actor state is defined in the global axis system.
      | The state is superponed on the Initial position defined in the GUI.
      |
      | For more information, please click Help.
      settings: OpenFcn=open_system([gcb '/Actuator'],'mask')
      mask Help: eval('openHelp(222)')
      mask Display: image(imread('State.png'))
  STATE_CarTrailer_SingleAxle_1_bus : Subsystem  Tag=actuator/StatePort  Priority=0  LoadFcn=load('PreScanStateActuatorData.mat')  mask(PreScan Sink Block: State){}
      mask help:
      | The Actor State contains a vector signal of size (9x1), containing the following signals:
      |
      | -  Position    	(x,y,z)             	[m]
      | -  Velocity    	(vx,vy,vz)         	[m/s]
      | -  Angles       	(Roll, Pitch, Yaw)	[rad]
      |
      | The Actor state is defined in the global axis system.
      | The state is superponed on the Initial position defined in the GUI.
      |
      | For more information, please click Help.
      settings: OpenFcn=open_system([gcb '/Actuator'],'mask')
      mask Help: eval('openHelp(222)')
      mask Display: image(imread('State.png'))
  STATE_ChessPlaneBox_1_bus : Subsystem  Tag=actuator/StatePort  Priority=0  LoadFcn=load('PreScanStateActuatorData.mat')  mask(PreScan Sink Block: State){}
      mask help:
      | The Actor State contains a vector signal of size (9x1), containing the following signals:
      |
      | -  Position    	(x,y,z)             	[m]
      | -  Velocity    	(vx,vy,vz)         	[m/s]
      | -  Angles       	(Roll, Pitch, Yaw)	[rad]
      |
      | The Actor state is defined in the global axis system.
      | The state is superponed on the Initial position defined in the GUI.
      |
      | For more information, please click Help.
      settings: OpenFcn=open_system([gcb '/Actuator'],'mask')
      mask Help: eval('openHelp(222)')
      mask Display: image(imread('State.png'))
  STATE_Citroen_C3_1_bus : Subsystem  Tag=actuator/StatePort  Priority=0  LoadFcn=load('PreScanStateActuatorData.mat')  mask(PreScan Sink Block: State){}
      mask help:
      | The Actor State contains a vector signal of size (9x1), containing the following signals:
      |
      | -  Position    	(x,y,z)             	[m]
      | -  Velocity    	(vx,vy,vz)         	[m/s]
      | -  Angles       	(Roll, Pitch, Yaw)	[rad]
      |
      | The Actor state is defined in the global axis system.
      | The state is superponed on the Initial position defined in the GUI.
      |
      | For more information, please click Help.
      settings: OpenFcn=open_system([gcb '/Actuator'],'mask')
      mask Help: eval('openHelp(222)')
      mask Display: image(imread('State.png'))
  STATE_Fiat_Bravo_1_bus : Subsystem  Tag=actuator/StatePort  Priority=0  LoadFcn=load('PreScanStateActuatorData.mat')  mask(PreScan Sink Block: State){}
      mask help:
      | The Actor State contains a vector signal of size (9x1), containing the following signals:
      |
      | -  Position    	(x,y,z)             	[m]
      | -  Velocity    	(vx,vy,vz)         	[m/s]
      | -  Angles       	(Roll, Pitch, Yaw)	[rad]
      |
      | The Actor state is defined in the global axis system.
      | The state is superponed on the Initial position defined in the GUI.
      |
      | For more information, please click Help.
      settings: OpenFcn=open_system([gcb '/Actuator'],'mask')
      mask Help: eval('openHelp(222)')
      mask Display: image(imread('State.png'))
  STATE_Ford_FocusWagon_1_bus : Subsystem  Tag=actuator/StatePort  Priority=0  LoadFcn=load('PreScanStateActuatorData.mat')  mask(PreScan Sink Block: State){}
      mask help:
      | The Actor State contains a vector signal of size (9x1), containing the following signals:
      |
      | -  Position    	(x,y,z)             	[m]
      | -  Velocity    	(vx,vy,vz)         	[m/s]
      | -  Angles       	(Roll, Pitch, Yaw)	[rad]
      |
      | The Actor state is defined in the global axis system.
      | The state is superponed on the Initial position defined in the GUI.
      |
      | For more information, please click Help.
      settings: OpenFcn=open_system([gcb '/Actuator'],'mask')
      mask Help: eval('openHelp(222)')
      mask Display: image(imread('State.png'))
  STATE_Male_Regular_BendingOver_1_bus : Subsystem  Tag=actuator/StatePort  Priority=0  LoadFcn=load('PreScanStateActuatorData.mat')  mask(PreScan Sink Block: State){}
      mask help:
      | The Actor State contains a vector signal of size (9x1), containing the following signals:
      |
      | -  Position    	(x,y,z)             	[m]
      | -  Velocity    	(vx,vy,vz)         	[m/s]
      | -  Angles       	(Roll, Pitch, Yaw)	[rad]
      |
      | The Actor state is defined in the global axis system.
      | The state is superponed on the Initial position defined in the GUI.
      |
      | For more information, please click Help.
      settings: OpenFcn=open_system([gcb '/Actuator'],'mask')
      mask Help: eval('openHelp(222)')
      mask Display: image(imread('State.png'))
  STATE_Male_Regular_LeaningBack_1_bus : Subsystem  Tag=actuator/StatePort  Priority=0  LoadFcn=load('PreScanStateActuatorData.mat')  mask(PreScan Sink Block: State){}
      mask help:
      | The Actor State contains a vector signal of size (9x1), containing the following signals:
      |
      | -  Position    	(x,y,z)             	[m]
      | -  Velocity    	(vx,vy,vz)         	[m/s]
      | -  Angles       	(Roll, Pitch, Yaw)	[rad]
      |
      | The Actor state is defined in the global axis system.
      | The state is superponed on the Initial position defined in the GUI.
      |
      | For more information, please click Help.
      settings: OpenFcn=open_system([gcb '/Actuator'],'mask')
      mask Help: eval('openHelp(222)')
      mask Display: image(imread('State.png'))
  STATE_Male_Regular_LeaningBack_2_bus : Subsystem  Tag=actuator/StatePort  Priority=0  LoadFcn=load('PreScanStateActuatorData.mat')  mask(PreScan Sink Block: State){}
      mask help:
      | The Actor State contains a vector signal of size (9x1), containing the following signals:
      |
      | -  Position    	(x,y,z)             	[m]
      | -  Velocity    	(vx,vy,vz)         	[m/s]
      | -  Angles       	(Roll, Pitch, Yaw)	[rad]
      |
      | The Actor state is defined in the global axis system.
      | The state is superponed on the Initial position defined in the GUI.
      |
      | For more information, please click Help.
      settings: OpenFcn=open_system([gcb '/Actuator'],'mask')
      mask Help: eval('openHelp(222)')
      mask Display: image(imread('State.png'))
  STATE_Male_Regular_Leaning_1_bus : Subsystem  Tag=actuator/StatePort  Priority=0  LoadFcn=load('PreScanStateActuatorData.mat')  mask(PreScan Sink Block: State){}
      mask help:
      | The Actor State contains a vector signal of size (9x1), containing the following signals:
      |
      | -  Position    	(x,y,z)             	[m]
      | -  Velocity    	(vx,vy,vz)         	[m/s]
      | -  Angles       	(Roll, Pitch, Yaw)	[rad]
      |
      | The Actor state is defined in the global axis system.
      | The state is superponed on the Initial position defined in the GUI.
      |
      | For more information, please click Help.
      settings: OpenFcn=open_system([gcb '/Actuator'],'mask')
      mask Help: eval('openHelp(222)')
      mask Display: image(imread('State.png'))
  STATE_Male_Regular_LyingDown_1_bus : Subsystem  Tag=actuator/StatePort  Priority=0  LoadFcn=load('PreScanStateActuatorData.mat')  mask(PreScan Sink Block: State){}
      mask help:
      | The Actor State contains a vector signal of size (9x1), containing the following signals:
      |
      | -  Position    	(x,y,z)             	[m]
      | -  Velocity    	(vx,vy,vz)         	[m/s]
      | -  Angles       	(Roll, Pitch, Yaw)	[rad]
      |
      | The Actor state is defined in the global axis system.
      | The state is superponed on the Initial position defined in the GUI.
      |
      | For more information, please click Help.
      settings: OpenFcn=open_system([gcb '/Actuator'],'mask')
      mask Help: eval('openHelp(222)')
      mask Display: image(imread('State.png'))
  STATE_Mazda_RX8_1_bus : Subsystem  Tag=actuator/StatePort  Priority=0  LoadFcn=load('PreScanStateActuatorData.mat')  mask(PreScan Sink Block: State){}
      mask help:
      | The Actor State contains a vector signal of size (9x1), containing the following signals:
      |
      | -  Position    	(x,y,z)             	[m]
      | -  Velocity    	(vx,vy,vz)         	[m/s]
      | -  Angles       	(Roll, Pitch, Yaw)	[rad]
      |
      | The Actor state is defined in the global axis system.
      | The state is superponed on the Initial position defined in the GUI.
      |
      | For more information, please click Help.
      settings: OpenFcn=open_system([gcb '/Actuator'],'mask')
      mask Help: eval('openHelp(222)')
      mask Display: image(imread('State.png'))
  STATE_Nissan_Cabstar_1_bus : Subsystem  Tag=actuator/StatePort  Priority=0  LoadFcn=load('PreScanStateActuatorData.mat')  mask(PreScan Sink Block: State){}
      mask help:
      | The Actor State contains a vector signal of size (9x1), containing the following signals:
      |
      | -  Position    	(x,y,z)             	[m]
      | -  Velocity    	(vx,vy,vz)         	[m/s]
      | -  Angles       	(Roll, Pitch, Yaw)	[rad]
      |
      | The Actor state is defined in the global axis system.
      | The state is superponed on the Initial position defined in the GUI.
      |
      | For more information, please click Help.
      settings: OpenFcn=open_system([gcb '/Actuator'],'mask')
      mask Help: eval('openHelp(222)')
      mask Display: image(imread('State.png'))
  STATE_Sphere_1_bus : Subsystem  Tag=actuator/StatePort  Priority=0  LoadFcn=load('PreScanStateActuatorData.mat')  mask(PreScan Sink Block: State){}
      mask help:
      | The Actor State contains a vector signal of size (9x1), containing the following signals:
      |
      | -  Position    	(x,y,z)             	[m]
      | -  Velocity    	(vx,vy,vz)         	[m/s]
      | -  Angles       	(Roll, Pitch, Yaw)	[rad]
      |
      | The Actor state is defined in the global axis system.
      | The state is superponed on the Initial position defined in the GUI.
      |
      | For more information, please click Help.
      settings: OpenFcn=open_system([gcb '/Actuator'],'mask')
      mask Help: eval('openHelp(222)')
      mask Display: image(imread('State.png'))
  STATE_Toyota_Previa_1_bus : Subsystem  Tag=actuator/StatePort  Priority=0  LoadFcn=load('PreScanStateActuatorData.mat')  mask(PreScan Sink Block: State){}
      mask help:
      | The Actor State contains a vector signal of size (9x1), containing the following signals:
      |
      | -  Position    	(x,y,z)             	[m]
      | -  Velocity    	(vx,vy,vz)         	[m/s]
      | -  Angles       	(Roll, Pitch, Yaw)	[rad]
      |
      | The Actor state is defined in the global axis system.
      | The state is superponed on the Initial position defined in the GUI.
      |
      | For more information, please click Help.
      settings: OpenFcn=open_system([gcb '/Actuator'],'mask')
      mask Help: eval('openHelp(222)')
      mask Display: image(imread('State.png'))
  STATE_Toyota_Yaris_1_bus : Subsystem  Tag=actuator/StatePort  Priority=0  LoadFcn=load('PreScanStateActuatorData.mat')  mask(PreScan Sink Block: State){}
      mask help:
      | The Actor State contains a vector signal of size (9x1), containing the following signals:
      |
      | -  Position    	(x,y,z)             	[m]
      | -  Velocity    	(vx,vy,vz)         	[m/s]
      | -  Angles       	(Roll, Pitch, Yaw)	[rad]
      |
      | The Actor state is defined in the global axis system.
      | The state is superponed on the Initial position defined in the GUI.
      |
      | For more information, please click Help.
      settings: OpenFcn=open_system([gcb '/Actuator'],'mask')
      mask Help: eval('openHelp(222)')
      mask Display: image(imread('State.png'))
  ScenarioEngine : Subsystem  Tag=PreScanOpenScenarioBlock  Priority=10  LoadFcn=load PrescanSynchronizeData  mask(PreScan Simulation Core Block){TimeStep=1/100}
      mask prompts: TimeStep "Timestep [s]"
      mask help:
      | Please do not remove this block from the PreScan compilation sheet,
      | as it contains essential configuration parameters for a PreScan simulation.
      settings: DeleteFcn=PreScanBlockDeleteFcn;
      mask Display: image(imread('prescanlogo.ico'))
  Sphere_1 : Subsystem  Tag=WorldObjectSubSystem  InitFcn=UniqueId = '3615';
      mask init:
      | imagePath=which('Sphere.jpg');
      mask Display: image(imread(imagePath));color('white');text(0, 0, ' ID=140\n')
  SteeringColumn_pivot_Audi_A8_1 : Subsystem  Tag=Actuator  Priority=0  LoadFcn=load('PrescanPoseData');load('PrescanXYZData');load('PreScanRPYData')
      mask help:
      | The VisuJoint block provides a way to adapt the location and orientation of a part of an object.
      |
      | For more information, please click Help.
      settings: OpenFcn=open_system([gcb '/Actuator'],'mask')
      mask Display: image(imread('Joint.png'))
  SteeringWheel_pivot_Audi_A8_1 : Subsystem  Tag=Actuator  Priority=0  LoadFcn=load('PrescanPoseData');load('PrescanXYZData');load('PreScanRPYData')
      mask help:
      | The VisuJoint block provides a way to adapt the location and orientation of a part of an object.
      |
      | For more information, please click Help.
      settings: OpenFcn=open_system([gcb '/Actuator'],'mask')
      mask Display: image(imread('Joint.png'))
  Synchronizer : Subsystem  Tag=PreScanSynchronizer  Priority=20  LoadFcn=load PrescanSynchronizeData  mask(PreScan Simulation Core Block){TimeStep=1/100}
      mask prompts: TimeStep "Timestep [s]"
      mask help:
      | Please do not remove this block from the PreScan compilation sheet,
      | as it contains essential configuration parameters for a PreScan simulation.
      settings: DeleteFcn=PreScanBlockDeleteFcn;
      mask Display: image(imread('prescanlogo.ico'))
  Toyota_Previa_1 : Subsystem  Tag=WorldObjectSubSystem  InitFcn=UniqueId = '3608';
      mask init:
      | modelPath = GenericModelHelper.getGenericModelFilePath('ModelDepo','Vehicles\Toyota_Previa\Toyota_Previa.pgmb','93e58f95175b34f6ce91a88cdfe55b40');imagePath = GenericModelHelper.getCompilationPicture(modelPath, 'Toyota_Previa_HighPoly.png');
      mask Display: image(imread(imagePath));color('white');text(0, 0, ' ID=138\n')
  Toyota_Yaris_1 : Subsystem  Tag=WorldObjectSubSystem  InitFcn=UniqueId = '3534';
      mask init:
      | modelPath = GenericModelHelper.getGenericModelFilePath('ModelDepo','Vehicles\Toyota_Yaris\Toyota_Yaris.pgmb','3ea2b9be97d70b5ca322b210574befd9');imagePath = GenericModelHelper.getCompilationPicture(modelPath, 'Toyota_Yaris_HighPoly.png');
      mask Display: image(imread(imagePath));color('white');text(0, 0, ' ID=132\n')
  V2X_Rx6115_CAM_Receiver : Subsystem  Tag=sensor/plugin/sfun_V2X_CAM_Receiver  Priority=30  mask(V2X CAM Receiver Block){}
      mask help: V2X Block receiving a CAM message
      settings: OpenFcn=open_system([gcb '/Sensor'],'mask')
      mask Help: eval('openHelp()')
      mask Display: image(imread('V2XR_grayscale.png'))
  V2X_Rx6115_DENM_Receiver : Subsystem  Tag=sensor/plugin/sfun_V2X_DENM_Receiver  Priority=30  mask(V2X DENM Receiver Block){}
      mask help: V2X Block receiving a DENM message
      settings: OpenFcn=open_system([gcb '/Sensor'],'mask')
      mask Help: eval('openHelp()')
      mask Display: image(imread('V2XR_grayscale.png'))
  V2X_Tx6114_CAM_Transmitter : Subsystem  Tag=actuator/plugin/sfun_V2X_CAM_Transmitter  Priority=0  mask(V2X CAM Transmitter Block){}
      mask help: V2X Block transmitting a CAM message
      settings: OpenFcn=open_system([gcb '/Actuator'],'mask')
      mask Help: eval('openHelp()')
      mask Display: image(imread('V2XT_grayscale.png'))
  V2X_Tx6114_DENM_Transmitter : Subsystem  Tag=actuator/plugin/sfun_V2X_DENM_Transmitter  Priority=0  mask(V2X DENM Transmitter Block){}
      mask help: V2X Block transmitting a DENM message
      settings: OpenFcn=open_system([gcb '/Actuator'],'mask')
      mask Help: eval('openHelp()')
      mask Display: image(imread('V2XT_grayscale.png'))
  V2X_Tx6193_CAM_Transmitter : Subsystem  Tag=actuator/plugin/sfun_V2X_CAM_Transmitter  Priority=0  mask(V2X CAM Transmitter Block){}
      mask help: V2X Block transmitting a CAM message
      settings: OpenFcn=open_system([gcb '/Actuator'],'mask')
      mask Help: eval('openHelp()')
      mask Display: image(imread('V2XT_grayscale.png'))
  V2X_Tx6193_DENM_Transmitter : Subsystem  Tag=actuator/plugin/sfun_V2X_DENM_Transmitter  Priority=0  mask(V2X DENM Transmitter Block){}
      mask help: V2X Block transmitting a DENM message
      settings: OpenFcn=open_system([gcb '/Actuator'],'mask')
      mask Help: eval('openHelp()')
      mask Display: image(imread('V2XT_grayscale.png'))
  V2X_Tx6194_CAM_Transmitter : Subsystem  Tag=actuator/plugin/sfun_V2X_CAM_Transmitter  Priority=0  mask(V2X CAM Transmitter Block){}
      mask help: V2X Block transmitting a CAM message
      settings: OpenFcn=open_system([gcb '/Actuator'],'mask')
      mask Help: eval('openHelp()')
      mask Display: image(imread('V2XT_grayscale.png'))
  V2X_Tx6194_DENM_Transmitter : Subsystem  Tag=actuator/plugin/sfun_V2X_DENM_Transmitter  Priority=0  mask(V2X DENM Transmitter Block){}
      mask help: V2X Block transmitting a DENM message
      settings: OpenFcn=open_system([gcb '/Actuator'],'mask')
      mask Help: eval('openHelp()')
      mask Display: image(imread('V2XT_grayscale.png'))
  V2X_Tx6195_CAM_Transmitter : Subsystem  Tag=actuator/plugin/sfun_V2X_CAM_Transmitter  Priority=0  mask(V2X CAM Transmitter Block){}
      mask help: V2X Block transmitting a CAM message
      settings: OpenFcn=open_system([gcb '/Actuator'],'mask')
      mask Help: eval('openHelp()')
      mask Display: image(imread('V2XT_grayscale.png'))
  V2X_Tx6195_DENM_Transmitter : Subsystem  Tag=actuator/plugin/sfun_V2X_DENM_Transmitter  Priority=0  mask(V2X DENM Transmitter Block){}
      mask help: V2X Block transmitting a DENM message
      settings: OpenFcn=open_system([gcb '/Actuator'],'mask')
      mask Help: eval('openHelp()')
      mask Display: image(imread('V2XT_grayscale.png'))
  V2X_Tx6196_CAM_Transmitter : Subsystem  Tag=actuator/plugin/sfun_V2X_CAM_Transmitter  Priority=0  mask(V2X CAM Transmitter Block){}
      mask help: V2X Block transmitting a CAM message
      settings: OpenFcn=open_system([gcb '/Actuator'],'mask')
      mask Help: eval('openHelp()')
      mask Display: image(imread('V2XT_grayscale.png'))
  V2X_Tx6196_DENM_Transmitter : Subsystem  Tag=actuator/plugin/sfun_V2X_DENM_Transmitter  Priority=0  mask(V2X DENM Transmitter Block){}
      mask help: V2X Block transmitting a DENM message
      settings: OpenFcn=open_system([gcb '/Actuator'],'mask')
      mask Help: eval('openHelp()')
      mask Display: image(imread('V2XT_grayscale.png'))
  V2X_Tx6197_CAM_Transmitter : Subsystem  Tag=actuator/plugin/sfun_V2X_CAM_Transmitter  Priority=0  mask(V2X CAM Transmitter Block){}
      mask help: V2X Block transmitting a CAM message
      settings: OpenFcn=open_system([gcb '/Actuator'],'mask')
      mask Help: eval('openHelp()')
      mask Display: image(imread('V2XT_grayscale.png'))
  V2X_Tx6197_DENM_Transmitter : Subsystem  Tag=actuator/plugin/sfun_V2X_DENM_Transmitter  Priority=0  mask(V2X DENM Transmitter Block){}
      mask help: V2X Block transmitting a DENM message
      settings: OpenFcn=open_system([gcb '/Actuator'],'mask')
      mask Help: eval('openHelp()')
      mask Display: image(imread('V2XT_grayscale.png'))
  V2X_Tx6198_CAM_Transmitter : Subsystem  Tag=actuator/plugin/sfun_V2X_CAM_Transmitter  Priority=0  mask(V2X CAM Transmitter Block){}
      mask help: V2X Block transmitting a CAM message
      settings: OpenFcn=open_system([gcb '/Actuator'],'mask')
      mask Help: eval('openHelp()')
      mask Display: image(imread('V2XT_grayscale.png'))
  V2X_Tx6198_DENM_Transmitter : Subsystem  Tag=actuator/plugin/sfun_V2X_DENM_Transmitter  Priority=0  mask(V2X DENM Transmitter Block){}
      mask help: V2X Block transmitting a DENM message
      settings: OpenFcn=open_system([gcb '/Actuator'],'mask')
      mask Help: eval('openHelp()')
      mask Display: image(imread('V2XT_grayscale.png'))
  V2X_Tx6199_CAM_Transmitter : Subsystem  Tag=actuator/plugin/sfun_V2X_CAM_Transmitter  Priority=0  mask(V2X CAM Transmitter Block){}
      mask help: V2X Block transmitting a CAM message
      settings: OpenFcn=open_system([gcb '/Actuator'],'mask')
      mask Help: eval('openHelp()')
      mask Display: image(imread('V2XT_grayscale.png'))
  V2X_Tx6199_DENM_Transmitter : Subsystem  Tag=actuator/plugin/sfun_V2X_DENM_Transmitter  Priority=0  mask(V2X DENM Transmitter Block){}
      mask help: V2X Block transmitting a DENM message
      settings: OpenFcn=open_system([gcb '/Actuator'],'mask')
      mask Help: eval('openHelp()')
      mask Display: image(imread('V2XT_grayscale.png'))
  V2X_Tx6200_CAM_Transmitter : Subsystem  Tag=actuator/plugin/sfun_V2X_CAM_Transmitter  Priority=0  mask(V2X CAM Transmitter Block){}
      mask help: V2X Block transmitting a CAM message
      settings: OpenFcn=open_system([gcb '/Actuator'],'mask')
      mask Help: eval('openHelp()')
      mask Display: image(imread('V2XT_grayscale.png'))
  V2X_Tx6200_DENM_Transmitter : Subsystem  Tag=actuator/plugin/sfun_V2X_DENM_Transmitter  Priority=0  mask(V2X DENM Transmitter Block){}
      mask help: V2X Block transmitting a DENM message
      settings: OpenFcn=open_system([gcb '/Actuator'],'mask')
      mask Help: eval('openHelp()')
      mask Display: image(imread('V2XT_grayscale.png'))
  V2X_Tx6201_CAM_Transmitter : Subsystem  Tag=actuator/plugin/sfun_V2X_CAM_Transmitter  Priority=0  mask(V2X CAM Transmitter Block){}
      mask help: V2X Block transmitting a CAM message
      settings: OpenFcn=open_system([gcb '/Actuator'],'mask')
      mask Help: eval('openHelp()')
      mask Display: image(imread('V2XT_grayscale.png'))
  V2X_Tx6201_DENM_Transmitter : Subsystem  Tag=actuator/plugin/sfun_V2X_DENM_Transmitter  Priority=0  mask(V2X DENM Transmitter Block){}
      mask help: V2X Block transmitting a DENM message
      settings: OpenFcn=open_system([gcb '/Actuator'],'mask')
      mask Help: eval('openHelp()')
      mask Display: image(imread('V2XT_grayscale.png'))
  V2X_Tx6202_CAM_Transmitter : Subsystem  Tag=actuator/plugin/sfun_V2X_CAM_Transmitter  Priority=0  mask(V2X CAM Transmitter Block){}
      mask help: V2X Block transmitting a CAM message
      settings: OpenFcn=open_system([gcb '/Actuator'],'mask')
      mask Help: eval('openHelp()')
      mask Display: image(imread('V2XT_grayscale.png'))
  V2X_Tx6202_DENM_Transmitter : Subsystem  Tag=actuator/plugin/sfun_V2X_DENM_Transmitter  Priority=0  mask(V2X DENM Transmitter Block){}
      mask help: V2X Block transmitting a DENM message
      settings: OpenFcn=open_system([gcb '/Actuator'],'mask')
      mask Help: eval('openHelp()')
      mask Display: image(imread('V2XT_grayscale.png'))
  VISUColorRegion_Lower_Body_Male_Regular_BendingOver_1 : Subsystem  Tag=actuator/ColorRegion  Priority=0  LoadFcn=load('PrescanColorData')  mask(PreScan Sink Block: VisuTextureColor){}
      mask help:
      | The VisuTextureColor block provides a way to adapt the color of a vehicle.
      |
      | For more information, please click Help.
      settings: OpenFcn=open_system([gcb '/Actuator'],'mask')
      mask Help: eval('openHelp(230)')
      mask Display: image(imread('TextureColor.png'))
  VISUColorRegion_Lower_Body_Male_Regular_LeaningBack_1 : Subsystem  Tag=actuator/ColorRegion  Priority=0  LoadFcn=load('PrescanColorData')  mask(PreScan Sink Block: VisuTextureColor){}
      mask help:
      | The VisuTextureColor block provides a way to adapt the color of a vehicle.
      |
      | For more information, please click Help.
      settings: OpenFcn=open_system([gcb '/Actuator'],'mask')
      mask Help: eval('openHelp(230)')
      mask Display: image(imread('TextureColor.png'))
  VISUColorRegion_Lower_Body_Male_Regular_LeaningBack_2 : Subsystem  Tag=actuator/ColorRegion  Priority=0  LoadFcn=load('PrescanColorData')  mask(PreScan Sink Block: VisuTextureColor){}
      mask help:
      | The VisuTextureColor block provides a way to adapt the color of a vehicle.
      |
      | For more information, please click Help.
      settings: OpenFcn=open_system([gcb '/Actuator'],'mask')
      mask Help: eval('openHelp(230)')
      mask Display: image(imread('TextureColor.png'))
  VISUColorRegion_Lower_Body_Male_Regular_Leaning_1 : Subsystem  Tag=actuator/ColorRegion  Priority=0  LoadFcn=load('PrescanColorData')  mask(PreScan Sink Block: VisuTextureColor){}
      mask help:
      | The VisuTextureColor block provides a way to adapt the color of a vehicle.
      |
      | For more information, please click Help.
      settings: OpenFcn=open_system([gcb '/Actuator'],'mask')
      mask Help: eval('openHelp(230)')
      mask Display: image(imread('TextureColor.png'))
  VISUColorRegion_Lower_Body_Male_Regular_LyingDown_1 : Subsystem  Tag=actuator/ColorRegion  Priority=0  LoadFcn=load('PrescanColorData')  mask(PreScan Sink Block: VisuTextureColor){}
      mask help:
      | The VisuTextureColor block provides a way to adapt the color of a vehicle.
      |
      | For more information, please click Help.
      settings: OpenFcn=open_system([gcb '/Actuator'],'mask')
      mask Help: eval('openHelp(230)')
      mask Display: image(imread('TextureColor.png'))
  VISUColorRegion_Shoes_Male_Regular_BendingOver_1 : Subsystem  Tag=actuator/ColorRegion  Priority=0  LoadFcn=load('PrescanColorData')  mask(PreScan Sink Block: VisuTextureColor){}
      mask help:
      | The VisuTextureColor block provides a way to adapt the color of a vehicle.
      |
      | For more information, please click Help.
      settings: OpenFcn=open_system([gcb '/Actuator'],'mask')
      mask Help: eval('openHelp(230)')
      mask Display: image(imread('TextureColor.png'))
  VISUColorRegion_Shoes_Male_Regular_LeaningBack_1 : Subsystem  Tag=actuator/ColorRegion  Priority=0  LoadFcn=load('PrescanColorData')  mask(PreScan Sink Block: VisuTextureColor){}
      mask help:
      | The VisuTextureColor block provides a way to adapt the color of a vehicle.
      |
      | For more information, please click Help.
      settings: OpenFcn=open_system([gcb '/Actuator'],'mask')
      mask Help: eval('openHelp(230)')
      mask Display: image(imread('TextureColor.png'))
  VISUColorRegion_Shoes_Male_Regular_LeaningBack_2 : Subsystem  Tag=actuator/ColorRegion  Priority=0  LoadFcn=load('PrescanColorData')  mask(PreScan Sink Block: VisuTextureColor){}
      mask help:
      | The VisuTextureColor block provides a way to adapt the color of a vehicle.
      |
      | For more information, please click Help.
      settings: OpenFcn=open_system([gcb '/Actuator'],'mask')
      mask Help: eval('openHelp(230)')
      mask Display: image(imread('TextureColor.png'))
  VISUColorRegion_Shoes_Male_Regular_Leaning_1 : Subsystem  Tag=actuator/ColorRegion  Priority=0  LoadFcn=load('PrescanColorData')  mask(PreScan Sink Block: VisuTextureColor){}
      mask help:
      | The VisuTextureColor block provides a way to adapt the color of a vehicle.
      |
      | For more information, please click Help.
      settings: OpenFcn=open_system([gcb '/Actuator'],'mask')
      mask Help: eval('openHelp(230)')
      mask Display: image(imread('TextureColor.png'))
  VISUColorRegion_Shoes_Male_Regular_LyingDown_1 : Subsystem  Tag=actuator/ColorRegion  Priority=0  LoadFcn=load('PrescanColorData')  mask(PreScan Sink Block: VisuTextureColor){}
      mask help:
      | The VisuTextureColor block provides a way to adapt the color of a vehicle.
      |
      | For more information, please click Help.
      settings: OpenFcn=open_system([gcb '/Actuator'],'mask')
      mask Help: eval('openHelp(230)')
      mask Display: image(imread('TextureColor.png'))
  VISUColorRegion_Upper_Body_Male_Regular_BendingOver_1 : Subsystem  Tag=actuator/ColorRegion  Priority=0  LoadFcn=load('PrescanColorData')  mask(PreScan Sink Block: VisuTextureColor){}
      mask help:
      | The VisuTextureColor block provides a way to adapt the color of a vehicle.
      |
      | For more information, please click Help.
      settings: OpenFcn=open_system([gcb '/Actuator'],'mask')
      mask Help: eval('openHelp(230)')
      mask Display: image(imread('TextureColor.png'))
  VISUColorRegion_Upper_Body_Male_Regular_LeaningBack_1 : Subsystem  Tag=actuator/ColorRegion  Priority=0  LoadFcn=load('PrescanColorData')  mask(PreScan Sink Block: VisuTextureColor){}
      mask help:
      | The VisuTextureColor block provides a way to adapt the color of a vehicle.
      |
      | For more information, please click Help.
      settings: OpenFcn=open_system([gcb '/Actuator'],'mask')
      mask Help: eval('openHelp(230)')
      mask Display: image(imread('TextureColor.png'))
  VISUColorRegion_Upper_Body_Male_Regular_LeaningBack_2 : Subsystem  Tag=actuator/ColorRegion  Priority=0  LoadFcn=load('PrescanColorData')  mask(PreScan Sink Block: VisuTextureColor){}
      mask help:
      | The VisuTextureColor block provides a way to adapt the color of a vehicle.
      |
      | For more information, please click Help.
      settings: OpenFcn=open_system([gcb '/Actuator'],'mask')
      mask Help: eval('openHelp(230)')
      mask Display: image(imread('TextureColor.png'))
  VISUColorRegion_Upper_Body_Male_Regular_Leaning_1 : Subsystem  Tag=actuator/ColorRegion  Priority=0  LoadFcn=load('PrescanColorData')  mask(PreScan Sink Block: VisuTextureColor){}
      mask help:
      | The VisuTextureColor block provides a way to adapt the color of a vehicle.
      |
      | For more information, please click Help.
      settings: OpenFcn=open_system([gcb '/Actuator'],'mask')
      mask Help: eval('openHelp(230)')
      mask Display: image(imread('TextureColor.png'))
  VISUColorRegion_Upper_Body_Male_Regular_LyingDown_1 : Subsystem  Tag=actuator/ColorRegion  Priority=0  LoadFcn=load('PrescanColorData')  mask(PreScan Sink Block: VisuTextureColor){}
      mask help:
      | The VisuTextureColor block provides a way to adapt the color of a vehicle.
      |
      | For more information, please click Help.
      settings: OpenFcn=open_system([gcb '/Actuator'],'mask')
      mask Help: eval('openHelp(230)')
      mask Display: image(imread('TextureColor.png'))
  WheelL0_Audi_A8_1 : Subsystem  Tag=Actuator  Priority=0  LoadFcn=load('PrescanPoseData');load('PrescanXYZData');load('PreScanRPYData')
      mask help:
      | The VisuJoint block provides a way to adapt the location and orientation of a part of an object.
      |
      | For more information, please click Help.
      settings: OpenFcn=open_system([gcb '/Actuator'],'mask')
      mask Display: image(imread('Joint.png'))
  WheelL1_Audi_A8_1 : Subsystem  Tag=Actuator  Priority=0  LoadFcn=load('PrescanPoseData');load('PrescanXYZData');load('PreScanRPYData')
      mask help:
      | The VisuJoint block provides a way to adapt the location and orientation of a part of an object.
      |
      | For more information, please click Help.
      settings: OpenFcn=open_system([gcb '/Actuator'],'mask')
      mask Display: image(imread('Joint.png'))
  WheelR0_Audi_A8_1 : Subsystem  Tag=Actuator  Priority=0  LoadFcn=load('PrescanPoseData');load('PrescanXYZData');load('PreScanRPYData')
      mask help:
      | The VisuJoint block provides a way to adapt the location and orientation of a part of an object.
      |
      | For more information, please click Help.
      settings: OpenFcn=open_system([gcb '/Actuator'],'mask')
      mask Display: image(imread('Joint.png'))
  WheelR1_Audi_A8_1 : Subsystem  Tag=Actuator  Priority=0  LoadFcn=load('PrescanPoseData');load('PrescanXYZData');load('PreScanRPYData')
      mask help:
      | The VisuJoint block provides a way to adapt the location and orientation of a part of an object.
      |
      | For more information, please click Help.
      settings: OpenFcn=open_system([gcb '/Actuator'],'mask')
      mask Display: image(imread('Joint.png'))
  wires:
  Actros_1860_1/1(STATE_Actros_1860_1_bus) -> STATE_Actros_1860_1_bus/1(STATE_Actros_1860_1_bus)
  Actros_1860_1/2(V2X_Tx6202_CAM_Transmitter) -> V2X_Tx6202_CAM_Transmitter/1(V2X_Tx6202_CAM_Transmitter)
  Actros_1860_1/3(V2X_Tx6202_DENM_Transmitter) -> V2X_Tx6202_DENM_Transmitter/1(V2X_Tx6202_DENM_Transmitter)
  SELF_Actros_1860_1/1(SELF_Actros_1860_1) -> Actros_1860_1/1(SELF_Actros_1860_1)
  Actros_2541_1/1(STATE_Actros_2541_1_bus) -> STATE_Actros_2541_1_bus/1(STATE_Actros_2541_1_bus)
  Actros_2541_1/2(V2X_Tx6201_CAM_Transmitter) -> V2X_Tx6201_CAM_Transmitter/1(V2X_Tx6201_CAM_Transmitter)
  Actros_2541_1/3(V2X_Tx6201_DENM_Transmitter) -> V2X_Tx6201_DENM_Transmitter/1(V2X_Tx6201_DENM_Transmitter)
  SELF_Actros_2541_1/1(SELF_Actros_2541_1) -> Actros_2541_1/1(SELF_Actros_2541_1)
  Audi_A8_1/1(STATE_Audi_A8_1_bus) -> STATE_Audi_A8_1_bus/1(STATE_Audi_A8_1_bus)
  Audi_A8_1/2(WheelL0_Audi_A8_1) -> WheelL0_Audi_A8_1/1(WheelL0_Audi_A8_1)
  Audi_A8_1/3(WheelL1_Audi_A8_1) -> WheelL1_Audi_A8_1/1(WheelL1_Audi_A8_1)
  Audi_A8_1/4(WheelR0_Audi_A8_1) -> WheelR0_Audi_A8_1/1(WheelR0_Audi_A8_1)
  Audi_A8_1/5(WheelR1_Audi_A8_1) -> WheelR1_Audi_A8_1/1(WheelR1_Audi_A8_1)
  Audi_A8_1/6(SteeringWheel_pivot_Audi_A8_1) -> SteeringWheel_pivot_Audi_A8_1/1(SteeringWheel_pivot_Audi_A8_1)
  Audi_A8_1/7(SteeringColumn_pivot_Audi_A8_1) -> SteeringColumn_pivot_Audi_A8_1/1(SteeringColumn_pivot_Audi_A8_1)
  Audi_A8_1/8(Audi_A8_1_Brake_light_left) -> Audi_A8_1_Brake_light_left/1(Audi_A8_1_Brake_light_left)
  Audi_A8_1/9(Audi_A8_1_Brake_light_right) -> Audi_A8_1_Brake_light_right/1(Audi_A8_1_Brake_light_right)
  Audi_A8_1/10(Audi_A8_1_Indicator_front_left) -> Audi_A8_1_Indicator_front_left/1(Audi_A8_1_Indicator_front_left)
  Audi_A8_1/11(Audi_A8_1_Indicator_rear_left) -> Audi_A8_1_Indicator_rear_left/1(Audi_A8_1_Indicator_rear_left)
  Audi_A8_1/12(Audi_A8_1_Indicator_front_right) -> Audi_A8_1_Indicator_front_right/1(Audi_A8_1_Indicator_front_right)
  Audi_A8_1/13(Audi_A8_1_Indicator_rear_right) -> Audi_A8_1_Indicator_rear_right/1(Audi_A8_1_Indicator_rear_right)
  SELF_Audi_A8_1/1(SELF_Audi_A8_1) -> Audi_A8_1/1(SELF_Audi_A8_1)
  V2X_Rx6115_CAM_Receiver/1(V2X_Rx6115_CAM_Receiver) -> Audi_A8_1/2(V2X_Rx6115_CAM_Receiver)
  V2X_Rx6115_DENM_Receiver/1(V2X_Rx6115_DENM_Receiver) -> Audi_A8_1/3(V2X_Rx6115_DENM_Receiver)
  BMW_X5_1/1(STATE_BMW_X5_1_bus) -> STATE_BMW_X5_1_bus/1(STATE_BMW_X5_1_bus)
  BMW_X5_1/2(V2X_Tx6193_CAM_Transmitter) -> V2X_Tx6193_CAM_Transmitter/1(V2X_Tx6193_CAM_Transmitter)
  BMW_X5_1/3(V2X_Tx6193_DENM_Transmitter) -> V2X_Tx6193_DENM_Transmitter/1(V2X_Tx6193_DENM_Transmitter)
  SELF_BMW_X5_1/1(SELF_BMW_X5_1) -> BMW_X5_1/1(SELF_BMW_X5_1)
  CarTrailer_SingleAxle_1/1(STATE_CarTrailer_SingleAxle_1_bus) -> STATE_CarTrailer_SingleAxle_1_bus/1(STATE_CarTrailer_SingleAxle_1_bus)
  CarTrailer_SingleAxle_1/2(V2X_Tx6114_CAM_Transmitter) -> V2X_Tx6114_CAM_Transmitter/1(V2X_Tx6114_CAM_Transmitter)
  CarTrailer_SingleAxle_1/3(V2X_Tx6114_DENM_Transmitter) -> V2X_Tx6114_DENM_Transmitter/1(V2X_Tx6114_DENM_Transmitter)
  SELF_CarTrailer_SingleAxle_1/1(SELF_CarTrailer_SingleAxle_1) -> CarTrailer_SingleAxle_1/1(SELF_CarTrailer_SingleAxle_1)
  ChessPlaneBox_1/1(STATE_ChessPlaneBox_1_bus) -> STATE_ChessPlaneBox_1_bus/1(STATE_ChessPlaneBox_1_bus)
  SELF_ChessPlaneBox_1/1(SELF_ChessPlaneBox_1) -> ChessPlaneBox_1/1(SELF_ChessPlaneBox_1)
  Citroen_C3_1/1(STATE_Citroen_C3_1_bus) -> STATE_Citroen_C3_1_bus/1(STATE_Citroen_C3_1_bus)
  Citroen_C3_1/2(V2X_Tx6195_CAM_Transmitter) -> V2X_Tx6195_CAM_Transmitter/1(V2X_Tx6195_CAM_Transmitter)
  Citroen_C3_1/3(V2X_Tx6195_DENM_Transmitter) -> V2X_Tx6195_DENM_Transmitter/1(V2X_Tx6195_DENM_Transmitter)
  SELF_Citroen_C3_1/1(SELF_Citroen_C3_1) -> Citroen_C3_1/1(SELF_Citroen_C3_1)
  Fiat_Bravo_1/1(STATE_Fiat_Bravo_1_bus) -> STATE_Fiat_Bravo_1_bus/1(STATE_Fiat_Bravo_1_bus)
  Fiat_Bravo_1/2(V2X_Tx6197_CAM_Transmitter) -> V2X_Tx6197_CAM_Transmitter/1(V2X_Tx6197_CAM_Transmitter)
  Fiat_Bravo_1/3(V2X_Tx6197_DENM_Transmitter) -> V2X_Tx6197_DENM_Transmitter/1(V2X_Tx6197_DENM_Transmitter)
  SELF_Fiat_Bravo_1/1(SELF_Fiat_Bravo_1) -> Fiat_Bravo_1/1(SELF_Fiat_Bravo_1)
  Ford_FocusWagon_1/1(STATE_Ford_FocusWagon_1_bus) -> STATE_Ford_FocusWagon_1_bus/1(STATE_Ford_FocusWagon_1_bus)
  Ford_FocusWagon_1/2(V2X_Tx6194_CAM_Transmitter) -> V2X_Tx6194_CAM_Transmitter/1(V2X_Tx6194_CAM_Transmitter)
  Ford_FocusWagon_1/3(V2X_Tx6194_DENM_Transmitter) -> V2X_Tx6194_DENM_Transmitter/1(V2X_Tx6194_DENM_Transmitter)
  SELF_Ford_FocusWagon_1/1(SELF_Ford_FocusWagon_1) -> Ford_FocusWagon_1/1(SELF_Ford_FocusWagon_1)
  Male_Regular_BendingOver_1/1(STATE_Male_Regular_BendingOver_1_bus) -> STATE_Male_Regular_BendingOver_1_bus/1(STATE_Male_Regular_BendingOver_1_bus)
  SELF_Male_Regular_BendingOver_1/1(SELF_Male_Regular_BendingOver_1) -> Male_Regular_BendingOver_1/1(SELF_Male_Regular_BendingOver_1)
  Male_Regular_LeaningBack_1/1(STATE_Male_Regular_LeaningBack_1_bus) -> STATE_Male_Regular_LeaningBack_1_bus/1(STATE_Male_Regular_LeaningBack_1_bus)
  SELF_Male_Regular_LeaningBack_1/1(SELF_Male_Regular_LeaningBack_1) -> Male_Regular_LeaningBack_1/1(SELF_Male_Regular_LeaningBack_1)
  Male_Regular_LeaningBack_2/1(STATE_Male_Regular_LeaningBack_2_bus) -> STATE_Male_Regular_LeaningBack_2_bus/1(STATE_Male_Regular_LeaningBack_2_bus)
  SELF_Male_Regular_LeaningBack_2/1(SELF_Male_Regular_LeaningBack_2) -> Male_Regular_LeaningBack_2/1(SELF_Male_Regular_LeaningBack_2)
  Male_Regular_Leaning_1/1(STATE_Male_Regular_Leaning_1_bus) -> STATE_Male_Regular_Leaning_1_bus/1(STATE_Male_Regular_Leaning_1_bus)
  SELF_Male_Regular_Leaning_1/1(SELF_Male_Regular_Leaning_1) -> Male_Regular_Leaning_1/1(SELF_Male_Regular_Leaning_1)
  Male_Regular_LyingDown_1/1(STATE_Male_Regular_LyingDown_1_bus) -> STATE_Male_Regular_LyingDown_1_bus/1(STATE_Male_Regular_LyingDown_1_bus)
  SELF_Male_Regular_LyingDown_1/1(SELF_Male_Regular_LyingDown_1) -> Male_Regular_LyingDown_1/1(SELF_Male_Regular_LyingDown_1)
  Mazda_RX8_1/1(STATE_Mazda_RX8_1_bus) -> STATE_Mazda_RX8_1_bus/1(STATE_Mazda_RX8_1_bus)
  Mazda_RX8_1/2(Mazda_RX8_1_Brake_light_center) -> Mazda_RX8_1_Brake_light_center/1(Mazda_RX8_1_Brake_light_center)
  Mazda_RX8_1/3(Mazda_RX8_1_Brake_light_left) -> Mazda_RX8_1_Brake_light_left/1(Mazda_RX8_1_Brake_light_left)
  Mazda_RX8_1/4(Mazda_RX8_1_Brake_light_right) -> Mazda_RX8_1_Brake_light_right/1(Mazda_RX8_1_Brake_light_right)
  Mazda_RX8_1/5(Mazda_RX8_1_Indicator_front_left) -> Mazda_RX8_1_Indicator_front_left/1(Mazda_RX8_1_Indicator_front_left)
  Mazda_RX8_1/6(Mazda_RX8_1_Indicator_side_left) -> Mazda_RX8_1_Indicator_side_left/1(Mazda_RX8_1_Indicator_side_left)
  Mazda_RX8_1/7(Mazda_RX8_1_Indicator_rear_left) -> Mazda_RX8_1_Indicator_rear_left/1(Mazda_RX8_1_Indicator_rear_left)
  Mazda_RX8_1/8(Mazda_RX8_1_Indicator_front_right) -> Mazda_RX8_1_Indicator_front_right/1(Mazda_RX8_1_Indicator_front_right)
  Mazda_RX8_1/9(Mazda_RX8_1_Indicator_side_right) -> Mazda_RX8_1_Indicator_side_right/1(Mazda_RX8_1_Indicator_side_right)
  Mazda_RX8_1/10(Mazda_RX8_1_Indicator_rear_right) -> Mazda_RX8_1_Indicator_rear_right/1(Mazda_RX8_1_Indicator_rear_right)
  Mazda_RX8_1/11(V2X_Tx6199_CAM_Transmitter) -> V2X_Tx6199_CAM_Transmitter/1(V2X_Tx6199_CAM_Transmitter)
  Mazda_RX8_1/12(V2X_Tx6199_DENM_Transmitter) -> V2X_Tx6199_DENM_Transmitter/1(V2X_Tx6199_DENM_Transmitter)
  SELF_Mazda_RX8_1/1(SELF_Mazda_RX8_1) -> Mazda_RX8_1/1(SELF_Mazda_RX8_1)
  Nissan_Cabstar_1/1(STATE_Nissan_Cabstar_1_bus) -> STATE_Nissan_Cabstar_1_bus/1(STATE_Nissan_Cabstar_1_bus)
  Nissan_Cabstar_1/2(V2X_Tx6198_CAM_Transmitter) -> V2X_Tx6198_CAM_Transmitter/1(V2X_Tx6198_CAM_Transmitter)
  Nissan_Cabstar_1/3(V2X_Tx6198_DENM_Transmitter) -> V2X_Tx6198_DENM_Transmitter/1(V2X_Tx6198_DENM_Transmitter)
  SELF_Nissan_Cabstar_1/1(SELF_Nissan_Cabstar_1) -> Nissan_Cabstar_1/1(SELF_Nissan_Cabstar_1)
  SELF_Sphere_1/1(SELF_Sphere_1) -> Sphere_1/1(SELF_Sphere_1)
  Sphere_1/1(STATE_Sphere_1_bus) -> STATE_Sphere_1_bus/1(STATE_Sphere_1_bus)
  SELF_Toyota_Previa_1/1(SELF_Toyota_Previa_1) -> Toyota_Previa_1/1(SELF_Toyota_Previa_1)
  Toyota_Previa_1/1(STATE_Toyota_Previa_1_bus) -> STATE_Toyota_Previa_1_bus/1(STATE_Toyota_Previa_1_bus)
  Toyota_Previa_1/2(V2X_Tx6200_CAM_Transmitter) -> V2X_Tx6200_CAM_Transmitter/1(V2X_Tx6200_CAM_Transmitter)
  Toyota_Previa_1/3(V2X_Tx6200_DENM_Transmitter) -> V2X_Tx6200_DENM_Transmitter/1(V2X_Tx6200_DENM_Transmitter)
  SELF_Toyota_Yaris_1/1(SELF_Toyota_Yaris_1) -> Toyota_Yaris_1/1(SELF_Toyota_Yaris_1)
  Toyota_Yaris_1/1(STATE_Toyota_Yaris_1_bus) -> STATE_Toyota_Yaris_1_bus/1(STATE_Toyota_Yaris_1_bus)
  Toyota_Yaris_1/2(V2X_Tx6196_CAM_Transmitter) -> V2X_Tx6196_CAM_Transmitter/1(V2X_Tx6196_CAM_Transmitter)
  Toyota_Yaris_1/3(V2X_Tx6196_DENM_Transmitter) -> V2X_Tx6196_DENM_Transmitter/1(V2X_Tx6196_DENM_Transmitter)
  Male_Regular_LyingDown_1/2(VISUColorRegion_Upper_Body_Male_Regular_LyingDown_1) -> VISUColorRegion_Upper_Body_Male_Regular_LyingDown_1/1(VISUColorRegion_Upper_Body_Male_Regular_LyingDown_1)
  Male_Regular_LyingDown_1/3(VISUColorRegion_Lower_Body_Male_Regular_LyingDown_1) -> VISUColorRegion_Lower_Body_Male_Regular_LyingDown_1/1(VISUColorRegion_Lower_Body_Male_Regular_LyingDown_1)
  Male_Regular_LyingDown_1/4(VISUColorRegion_Shoes_Male_Regular_LyingDown_1) -> VISUColorRegion_Shoes_Male_Regular_LyingDown_1/1(VISUColorRegion_Shoes_Male_Regular_LyingDown_1)
  Male_Regular_BendingOver_1/2(VISUColorRegion_Upper_Body_Male_Regular_BendingOver_1) -> VISUColorRegion_Upper_Body_Male_Regular_BendingOver_1/1(VISUColorRegion_Upper_Body_Male_Regular_BendingOver_1)
  Male_Regular_BendingOver_1/3(VISUColorRegion_Lower_Body_Male_Regular_BendingOver_1) -> VISUColorRegion_Lower_Body_Male_Regular_BendingOver_1/1(VISUColorRegion_Lower_Body_Male_Regular_BendingOver_1)
  Male_Regular_BendingOver_1/4(VISUColorRegion_Shoes_Male_Regular_BendingOver_1) -> VISUColorRegion_Shoes_Male_Regular_BendingOver_1/1(VISUColorRegion_Shoes_Male_Regular_BendingOver_1)
  Male_Regular_Leaning_1/2(VISUColorRegion_Upper_Body_Male_Regular_Leaning_1) -> VISUColorRegion_Upper_Body_Male_Regular_Leaning_1/1(VISUColorRegion_Upper_Body_Male_Regular_Leaning_1)
  Male_Regular_Leaning_1/3(VISUColorRegion_Lower_Body_Male_Regular_Leaning_1) -> VISUColorRegion_Lower_Body_Male_Regular_Leaning_1/1(VISUColorRegion_Lower_Body_Male_Regular_Leaning_1)
  Male_Regular_Leaning_1/4(VISUColorRegion_Shoes_Male_Regular_Leaning_1) -> VISUColorRegion_Shoes_Male_Regular_Leaning_1/1(VISUColorRegion_Shoes_Male_Regular_Leaning_1)
  Male_Regular_LeaningBack_1/2(VISUColorRegion_Upper_Body_Male_Regular_LeaningBack_1) -> VISUColorRegion_Upper_Body_Male_Regular_LeaningBack_1/1(VISUColorRegion_Upper_Body_Male_Regular_LeaningBack_1)
  Male_Regular_LeaningBack_1/3(VISUColorRegion_Lower_Body_Male_Regular_LeaningBack_1) -> VISUColorRegion_Lower_Body_Male_Regular_LeaningBack_1/1(VISUColorRegion_Lower_Body_Male_Regular_LeaningBack_1)
  Male_Regular_LeaningBack_1/4(VISUColorRegion_Shoes_Male_Regular_LeaningBack_1) -> VISUColorRegion_Shoes_Male_Regular_LeaningBack_1/1(VISUColorRegion_Shoes_Male_Regular_LeaningBack_1)
  Male_Regular_LeaningBack_2/2(VISUColorRegion_Upper_Body_Male_Regular_LeaningBack_2) -> VISUColorRegion_Upper_Body_Male_Regular_LeaningBack_2/1(VISUColorRegion_Upper_Body_Male_Regular_LeaningBack_2)
  Male_Regular_LeaningBack_2/3(VISUColorRegion_Lower_Body_Male_Regular_LeaningBack_2) -> VISUColorRegion_Lower_Body_Male_Regular_LeaningBack_2/1(VISUColorRegion_Lower_Body_Male_Regular_LeaningBack_2)
  Male_Regular_LeaningBack_2/4(VISUColorRegion_Shoes_Male_Regular_LeaningBack_2) -> VISUColorRegion_Shoes_Male_Regular_LeaningBack_2/1(VISUColorRegion_Shoes_Male_Regular_LeaningBack_2)
